simulink model "F14_breach"  (R2020a)
settings: Solver=ode45  StartTime=0.0  StopTime=tspan(end)  RelTol=1e-4  AbsTol=1e-6
model workspace (MATLAB code in the model file + MAT data in the model file):
  Beta = 426.4352
  Gamma = 0.01
  Ka = 0.677
  Kf = -1.746
  Ki = -3.864
  Kq = 0.8156
  Md = -6.8847
  Mq = -0.6571
  Mw = -0.00592
  Sa = 0.005236
  Swg = 3
  Ta = 0.05
  Tal = 0.3959
  Ts = 0.1
  Uo = 689.4
  Vto = 690.4
  W1 = 2.971
  W2 = 4.144
  Wa = 10
  Zd = -63.9979
  Zw = -0.6385
  a = 2.5348
  b = 64.13
  cmdgain = 0.0349095447273
  g = 32.2
  other statements: f14dat
libraries: simulink x1
Description:
  | F-14 Longitudinal Flight Control (Updated)
  | 
  | This demonstration models a flight control for the longitudinal motion of a Grumman Aerospace
  | F-14 Tomcat.  First order linear approximations of the aircraft and actuator behavior are connected
  | to an analog flight control design that uses the pilot's stick pitch command as the set point for the
  | aircraft's pitch attitude and uses aircraft pitch angle and pitch rate to determine commands.   A
  | simplified Dryden wind gust model is incorporated to perturb the system.
  | 
  | Some updates to the original f14.mdl file included in this version:
  | 
  | The model scope for viewing signals, Scope1, was created using the Signal and Scope Manager
  | from the Tools menu.  The Signal and Scope Manager allows you to instrument your model
  | without having to add blocks to the model.  If you close a model scope, such as for batch
  | simulations, you can later reopen it by double-clicking the "scope" icon on the signal of
  | interest.
  | 
  | Parameters for the model are stored in a file named f14dat.m.  This file is loaded by the model
  | into the model workspace.  You can view and edit data in the model workspace directly by
  | using the Model Explorer, which is launched using the View/Model Explorer menu item or by
  | launching it from the Model Explorer toolbar button in the Simulink editor.
settings Model: FPTRunName=Active  ExtModeTrigMode=oneshot  ExtModeArmWhenConnect=off  ExtModeAutoUpdateStatusClock=off  Creator=The MathWorks, Inc.  LastModifiedBy=nikhil
settings SolverCC: AutoScaleAbsTol=off
settings DataIOCC: ExternalInput=[t__, u__]  InitialState=[]  LoadExternalInput=on  SaveFormat=StructureWithTime  SaveState=on
settings OptimizationCC: BlockReduction=off  BooleanDataType=off  ConditionallyExecuteInputs=off  BufferReuse=off  GlobalBufferReuse=off  ExpressionDepthLimit=2147483647  LocalBlockOutputs=off  InitFltsAndDblsToZero=on  LifeSpan=inf  BufferReusableBoundary=off  SimCompilerOptimization=on  OptimizeDataStoreBuffers=off  BusAssignmentInplaceUpdate=off
settings DebuggingCC: SaveWithParameterizedLinksMsg=none  SignalResolutionControl=TryResolveAllWithWarning  MultiTaskDSMMsg=warning  MultiTaskCondExecSysMsg=none  IntegerOverflowMsg=none  FcnCallInpInsideContextMsg=warning  StateNameClashWarn=warning  SFUnexpectedBacktrackingDiag=warning  SFNoUnconditionalDefaultTransitionDiag=warning  SFExecutionAtInitializationDiag=none  IntegerSaturationMsg=none  ArithmeticOperatorsInVariantConditions=warning
settings HardwareCC: ProdBitPerPointer=32  ProdBitPerSizeT=32  ProdBitPerPtrDiffT=32  ProdLargestAtomicFloat=None  ProdIntDivRoundTo=Undefined  ProdEndianess=Unspecified  ProdWordSize=32  ProdHWDeviceType=32-bit Generic  TargetUnknown=on
settings ModelReferenceCC: PropagateSignalLabelsOutOfModel=off
settings SFSimCC: SimUseLocalCustomCode=off  CustomCodeUndefinedFunction=UseInterfaceOnly
settings RTWCC: Description=Generic Real-Time Target  RTWUseLocalCustomCode=off
settings CodeAppCC: StateflowObjectComments=on
settings GRTTargetCC: TargetFcnLib=ansi_tfl_tmw.mat  TargetLangStandard=C89/C90 (ANSI)  CombineOutputUpdateFcns=off  GRTInterface=on
settings ConfigComp: CovMetricSettings=dw  CovHtmlReporting=on  CovSaveCumulativeToWorkspaceVar=on  CovSaveSingleToWorkspaceVar=on  CovExternalEMLEnable=off  CovSFcnEnable=off

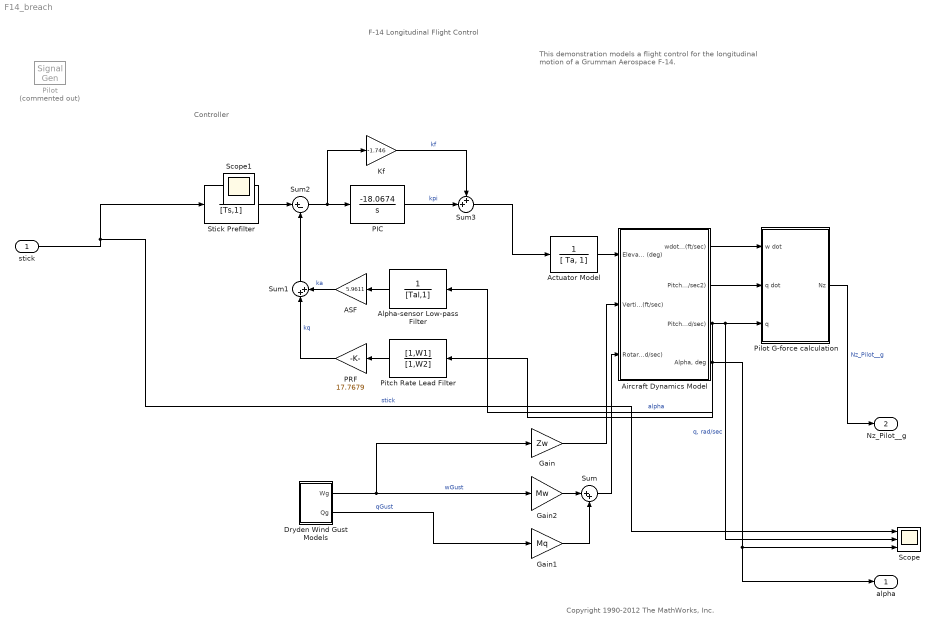
== system F14_breach ==
  note: Controller
  note: F-14 Longitudinal Flight Control
  note: This demonstration models a flight control
      | for the longitudinal motion of a Grumman Aerospace F-14.
  note: Copyright 1990-2012 The MathWorks, Inc.
  stick : Inport
  ASF : Gain  Gain=5.9611  SaturateOnIntegerOverflow=on  OutDataTypeStr=Inherit: Same as input  ParamDataTypeStr=Inherit: Same as input
  Actuator Model : TransferFcn  Denominator=[ Ta, 1]
  Aircraft Dynamics Model : Subsystem
      mask Display:
      | port_label('input',1,'\delta_{e}, deg','texmode','on');
      | port_label('input',2,'wGust, ft/sec','texmode','on');
      | port_label('input',3,'qGust, rad/sec','texmode','on');
      | port_label('output',1,'w, ft/sec','texmode','on');
      | port_label('output',2,'qdot, rad/sec^{2}','texmode','on');
      | port_label('output',3,'q, rad/sec','texmode','on');
      | port_label('output',4,'\alpha, rad','texmode','on');
  Alpha-sensor Low-pass Filter : TransferFcn  Denominator=[Tal,1]
  Dryden Wind Gust Models : Subsystem
      mask Display:
      | port_label('output',1,'wg','texmode','on');
      | port_label('output',2,'qg','texmode','on');
  Gain : Gain  Gain=Zw  SaturateOnIntegerOverflow=on  OutDataTypeStr=Inherit: Same as input  ParamDataTypeStr=Inherit: Same as input
  Gain1 : Gain  Gain=Mq  SaturateOnIntegerOverflow=on  OutDataTypeStr=Inherit: Same as input  ParamDataTypeStr=Inherit: Same as input
  Gain2 : Gain  Gain=Mw  SaturateOnIntegerOverflow=on  OutDataTypeStr=Inherit: Same as input  ParamDataTypeStr=Inherit: Same as input
  Kf : Gain  Gain=-1.746  SaturateOnIntegerOverflow=on  OutDataTypeStr=Inherit: Same as input  ParamDataTypeStr=Inherit: Same as input
  PIC : TransferFcn  Numerator=-18.0674  Denominator=[1 0]
  PRF : Gain  Gain=17.7679  SaturateOnIntegerOverflow=on  OutDataTypeStr=Inherit: Same as input  ParamDataTypeStr=Inherit: Same as input
  Pilot : SignalGenerator  Commented=on  WaveForm=square  Amplitude=0.5  Frequency=0.500000  Units=rad/sec
  Pilot G-force calculation : Subsystem
      mask Display:
      | port_label('input',1,'w, ft/sec','texmode','on');
      | port_label('input',2,'qdot','texmode','on');
      | port_label('input',3,'q, rad/sec','texmode','on');
      | port_label('output',1,'NzPilot, g','texmode','on');
  Pitch Rate Lead Filter : TransferFcn  Numerator=[1,W1]  Denominator=[1,W2]
  Scope : Scope  NumInputPorts=3
  Stick Prefilter : TransferFcn  Denominator=[Ts,1]
  Sum : Sum  Inputs=|++  InputSameDT=on  SaturateOnIntegerOverflow=on  OutDataTypeStr=Inherit: Same as first input
  Sum1 : Sum  Inputs=|++  InputSameDT=on  SaturateOnIntegerOverflow=on  OutDataTypeStr=Inherit: Same as first input
  Sum2 : Sum  Inputs=|+-  InputSameDT=on  SaturateOnIntegerOverflow=on  OutDataTypeStr=Inherit: Same as first input
  Sum3 : Sum  Inputs=++|  InputSameDT=on  SaturateOnIntegerOverflow=on  OutDataTypeStr=Inherit: Same as first input
  alpha : Outport  InitialOutput=0  VectorParamsAs1DForOutWhenUnconnected=off
  Nz_Pilot__g : Outport  Port=2  InitialOutput=0  VectorParamsAs1DForOutWhenUnconnected=off
  Scope1 : Scope
  wires:
  Pilot G-force calculation/1(Nz) -> Nz_Pilot__g/1  "Nz_Pilot__g"
  Gain2/1 -> Sum/1
  Gain/1 -> Aircraft Dynamics Model/2(Vertical Gust wGust (ft/sec))
  Dryden Wind Gust Models/2(Qg) -> Gain1/1  "qGust"
  Dryden Wind Gust Models/1(Wg) -> Gain2/1, Gain/1  "wGust"
  Sum/1 -> Aircraft Dynamics Model/3(Rotary Gust qGust (rad/sec))
  Gain1/1 -> Sum/2
  Actuator Model/1 -> Aircraft Dynamics Model/1(Elevator Deflection d (deg))
  Sum3/1 -> Actuator Model/1
  stick/1 -> Stick Prefilter/1, Scope/1  "stick"
  Aircraft Dynamics Model/1(wdot (ft/sec)) -> Pilot G-force calculation/1(w dot)
  Aircraft Dynamics Model/2(Pitch Accel qdot (rad/sec2)) -> Pilot G-force calculation/2(q dot)
  Aircraft Dynamics Model/3(Pitch Rate q (rad/sec)) -> Scope/2, Pilot G-force calculation/3(q), Pitch Rate Lead Filter/1  "q, rad/sec"
  Aircraft Dynamics Model/4("Alpha, deg") -> Scope/3, alpha/1, Alpha-sensor Low-pass Filter/1  "alpha"
  Alpha-sensor Low-pass Filter/1 -> ASF/1
  Pitch Rate Lead Filter/1 -> PRF/1
  Sum1/1 -> Sum2/2
  ASF/1 -> Sum1/2  "ka"
  PRF/1 -> Sum1/1  "kq"
  Stick Prefilter/1 -> Sum2/1
  PIC/1 -> Sum3/2  "kpi"
  Kf/1 -> Sum3/1  "kf"
  Sum2/1 -> PIC/1, Kf/1

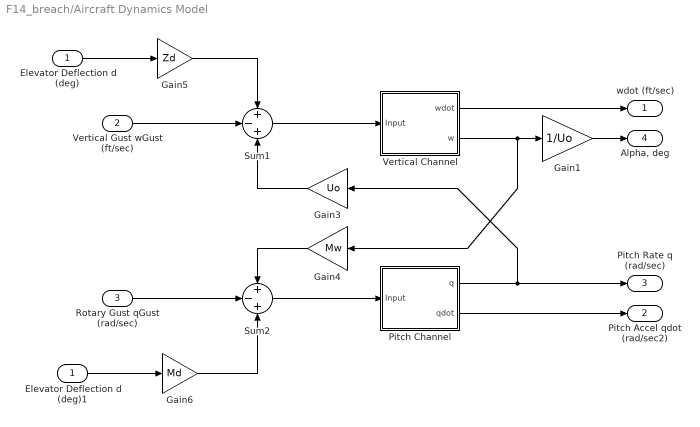
== system F14_breach/Aircraft Dynamics Model ==
  Elevator Deflection d (deg) : Inport
  Vertical Gust wGust (ft/sec) : Inport  Port=2
  Rotary Gust qGust (rad/sec) : Inport  Port=3
  Elevator Deflection d (deg)1 : InportShadow
  Gain1 : Gain  Gain=1/Uo  SaturateOnIntegerOverflow=on  OutDataTypeStr=Inherit: Same as input  ParamDataTypeStr=Inherit: Same as input
  Gain3 : Gain  Gain=Uo  SaturateOnIntegerOverflow=on  OutDataTypeStr=Inherit: Same as input  ParamDataTypeStr=Inherit: Same as input
  Gain4 : Gain  Gain=Mw  SaturateOnIntegerOverflow=on  OutDataTypeStr=Inherit: Same as input  ParamDataTypeStr=Inherit: Same as input
  Gain5 : Gain  Gain=Zd  SaturateOnIntegerOverflow=on  OutDataTypeStr=Inherit: Same as input  ParamDataTypeStr=Inherit: Same as input
  Gain6 : Gain  Gain=Md  SaturateOnIntegerOverflow=on  OutDataTypeStr=Inherit: Same as input  ParamDataTypeStr=Inherit: Same as input
  Pitch Channel : Subsystem
  Sum1 : Sum  Inputs=+-+  InputSameDT=on  SaturateOnIntegerOverflow=on  OutDataTypeStr=Inherit: Same as first input
  Sum2 : Sum  Inputs=+-+  InputSameDT=on  SaturateOnIntegerOverflow=on  OutDataTypeStr=Inherit: Same as first input
  Vertical Channel : Subsystem
  wdot (ft/sec) : Outport  InitialOutput=0  VectorParamsAs1DForOutWhenUnconnected=off
  Pitch Accel qdot (rad/sec2) : Outport  Port=2  InitialOutput=0  VectorParamsAs1DForOutWhenUnconnected=off
  Pitch Rate q (rad/sec) : Outport  Port=3  InitialOutput=0  VectorParamsAs1DForOutWhenUnconnected=off
  "Alpha, deg" : Outport  Port=4  InitialOutput=0  VectorParamsAs1DForOutWhenUnconnected=off
  wires:
  Vertical Channel/2(w) -> Gain4/1, Gain1/1
  Pitch Channel/1(q) -> Pitch Rate q (rad/sec)/1, Gain3/1
  Gain6/1 -> Sum2/3
  Gain5/1 -> Sum1/1
  Gain3/1 -> Sum1/3
  Rotary Gust qGust (rad/sec)/1 -> Sum2/2
  Sum2/1 -> Pitch Channel/1(Input)
  Sum1/1 -> Vertical Channel/1(Input)
  Gain4/1 -> Sum2/1
  Vertical Gust wGust (ft/sec)/1 -> Sum1/2
  Elevator Deflection d (deg)/1 -> Gain5/1
  Elevator Deflection d (deg)1/1 -> Gain6/1
  Gain1/1 -> "Alpha, deg"/1
  Vertical Channel/1(wdot) -> wdot (ft/sec)/1
  Pitch Channel/2(qdot) -> Pitch Accel qdot (rad/sec2)/1

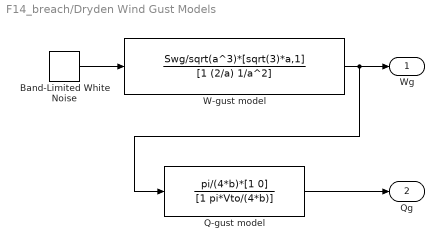
== system F14_breach/Dryden Wind Gust Models ==
  Band-Limited White Noise : simulink/Sources/Band-Limited White Noise  Cov=1  Ts=0.1  seed=[23341]
  Q-gust model : TransferFcn  Numerator=pi/(4*b)*[1 0]  Denominator=[1 pi*Vto/(4*b)]
  W-gust model : TransferFcn  Numerator=Swg/sqrt(a^3)*[sqrt(3)*a,1]  Denominator=[1 (2/a) 1/a^2]
  Wg : Outport  InitialOutput=0  VectorParamsAs1DForOutWhenUnconnected=off
  Qg : Outport  Port=2  InitialOutput=0  VectorParamsAs1DForOutWhenUnconnected=off
  wires:
  Band-Limited White Noise/1 -> W-gust model/1
  Q-gust model/1 -> Qg/1
  W-gust model/1 -> Wg/1, Q-gust model/1

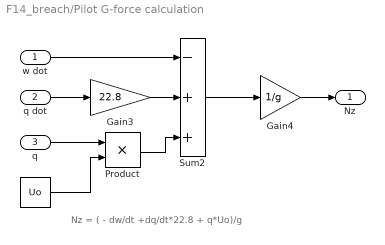
== system F14_breach/Pilot G-force calculation ==
  note: Nz = ( - dw/dt +dq/dt*22.8 + q*Uo)/g
  w dot : Inport
  q dot : Inport  Port=2
  q : Inport  Port=3
  " " : Constant  Value=Uo
  Gain3 : Gain  Gain=22.8  SaturateOnIntegerOverflow=on  OutDataTypeStr=Inherit: Same as input  ParamDataTypeStr=Inherit: Same as input
  Gain4 : Gain  Gain=1/g  SaturateOnIntegerOverflow=on  OutDataTypeStr=Inherit: Same as input  ParamDataTypeStr=Inherit: Same as input
  Product : Product  InputSameDT=on  RndMeth=Zero  SaturateOnIntegerOverflow=on  OutDataTypeStr=Inherit: Same as first input
  Sum2 : Sum  Inputs=-++  InputSameDT=on  SaturateOnIntegerOverflow=on  OutDataTypeStr=Inherit: Same as first input
  Nz : Outport  InitialOutput=0  VectorParamsAs1DForOutWhenUnconnected=off
  wires:
  Sum2/1 -> Gain4/1
  w dot/1 -> Sum2/1
  Gain4/1 -> Nz/1
  q dot/1 -> Gain3/1
  Gain3/1 -> Sum2/2
  Product/1 -> Sum2/3
  q/1 -> Product/1
  " "/1 -> Product/2

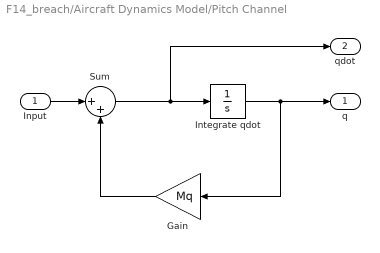
== system F14_breach/Aircraft Dynamics Model/Pitch Channel ==
  Input : Inport
  Gain : Gain  Gain=Mq  SaturateOnIntegerOverflow=on  OutDataTypeStr=Inherit: Same as input  ParamDataTypeStr=Inherit: Same as input
  Integrate qdot : Integrator
  Sum : Sum  Inputs=|++  InputSameDT=on  SaturateOnIntegerOverflow=on  OutDataTypeStr=Inherit: Same as first input
  q : Outport  InitialOutput=0  VectorParamsAs1DForOutWhenUnconnected=off
  qdot : Outport  Port=2  InitialOutput=0  VectorParamsAs1DForOutWhenUnconnected=off
  wires:
  Sum/1 -> qdot/1, Integrate qdot/1
  Integrate qdot/1 -> Gain/1, q/1
  Gain/1 -> Sum/2
  Input/1 -> Sum/1

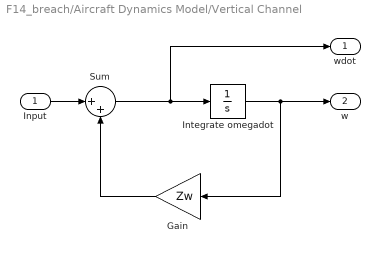
== system F14_breach/Aircraft Dynamics Model/Vertical Channel ==
  Input : Inport
  Gain : Gain  Gain=Zw  SaturateOnIntegerOverflow=on  OutDataTypeStr=Inherit: Same as input  ParamDataTypeStr=Inherit: Same as input
  Integrate omegadot : Integrator
  Sum : Sum  Inputs=|++  InputSameDT=on  SaturateOnIntegerOverflow=on  OutDataTypeStr=Inherit: Same as first input
  wdot : Outport  InitialOutput=0  VectorParamsAs1DForOutWhenUnconnected=off
  w : Outport  Port=2  InitialOutput=0  VectorParamsAs1DForOutWhenUnconnected=off
  wires:
  Input/1 -> Sum/1
  Gain/1 -> Sum/2
  Integrate omegadot/1 -> w/1, Gain/1
  Sum/1 -> Integrate omegadot/1, wdot/1
